simulink model "sist2"  (R2013b)
settings: Solver=ode45  StartTime=0.0  StopTime=10.0  RelTol=1e-3
settings Model: Creator=juan_  LastModifiedBy=juan_

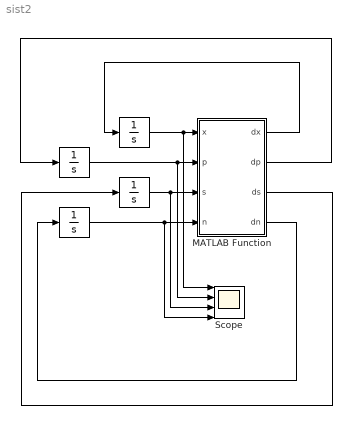
== system sist2 ==
  " " : Integrator
  "  " : Integrator
  " " : Integrator
  "    " : Integrator
  MATLAB Function : MATLAB Function  TreatAsAtomicUnit=on
  Scope : Scope  NumInputPorts=4
      settings: YMin=-5~-5~-5~-5  YMax=5~5~5~5
  wires:
  " "/1 -> Scope/1, MATLAB Function/1(x)
  "  "/1 -> Scope/3, MATLAB Function/3(s)
  "    "/1 -> Scope/4, MATLAB Function/4(n)
  MATLAB Function/1(dx) -> " "/1
  MATLAB Function/3(ds) -> "  "/1
  MATLAB Function/4(dn) -> "    "/1
  " "/1 -> Scope/2, MATLAB Function/2(p)
  MATLAB Function/2(dp) -> " "/1

== matlab function sist2/MATLAB Function ==
  data: x input; p input; dx output; dp output; s input; n input; ds output; dn output
function [dx,dp,ds,dn] = fcn(x,p,s,n)

%especificos del proceso:
k_s1=1/0.48;
k_s2=1/0.3;
k_n=1/8.9;
k_p1=0.0657;

%depende de la alimentacion, configurado en script:
%s_in=25;
%n_in=5;

%valores iniciales, van en los bloques integradores:
%{
x0=1;
p0=0;
s0=50;
n0=5;
%}

%constantes para modelos cineticos:
u_max=0.46;
K_s=1.2;
K_is=16.728;
K_n=0.254;
K_in=1.5;
q_pmax=0.126;
K_ps=4.1;
K_ips=80;
K_ipn=0.262;

%modelos cineticos:
rx=x*u_max*(s/(K_s+s+(s^2/(K_is))))*(n/(K_n+n));

rp=x*q_pmax*s/(K_ps + s + s^2/K_ips);
rp=rp*K_ipn/(K_ipn + n);
rp=rp+k_p1*rx;

rs=-(k_s1*rx + k_s2*rp);
rn=-k_n*rx;

dx= rx+D*(-x);
dp=rp+D*(-p);
ds= rs+D*(s_in-s);
dn= rn+D*(n_in-n);
